simulink model "model_1D_jumpup"  (R2016a)
settings: Solver=FixedStepAuto  StartTime=0.0  StopTime=10.0  FixedStep=deltaT  RelTol=1e-3
undefined symbols (not defined in the file): C_phi, g, l_AB, l_AC, m_K, m_R, O_A_K, phi_0, phi__d_0
settings Model: Creator=ich  LastModifiedBy=ich

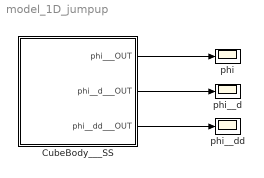
== system model_1D_jumpup ==
  CubeBody___SS : Subsystem
  phi : Scope
  phi__d : Scope
  phi__dd : Scope
  wires:
  CubeBody___SS/3(phi__dd___OUT) -> phi__dd/1
  CubeBody___SS/1(phi___OUT) -> phi/1
  CubeBody___SS/2(phi__d___OUT) -> phi__d/1

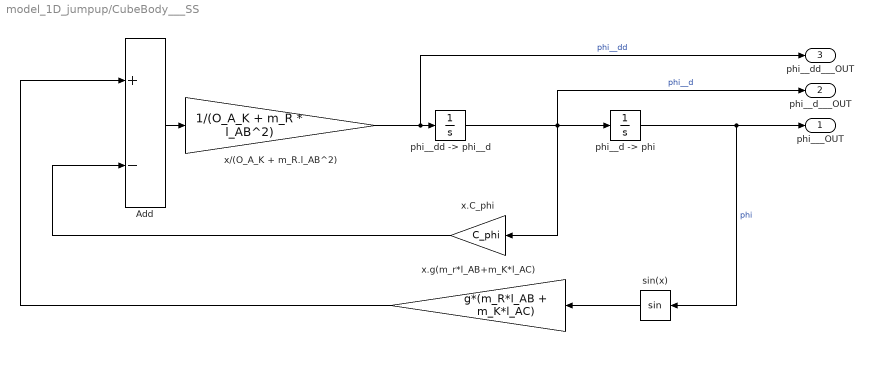
== system model_1D_jumpup/CubeBody___SS ==
  Add : Sum  Inputs=+-
  "phi__d -> phi" : Integrator  InitialCondition=phi_0
  "phi__dd -> phi__d" : Integrator  InitialCondition=phi__d_0
  sin(x) : Trigonometry
  x.C_phi : Gain  Gain=C_phi
  x.g(m_r*l_AB+m_K*l_AC) : Gain  Gain=g*(m_R*l_AB + m_K*l_AC)
  x/(O_A_K + m_R.l_AB^2) : Gain  Gain=1/(O_A_K + m_R * l_AB^2)
  phi___OUT : Outport
  phi__d___OUT : Outport  Port=2
  phi__dd___OUT : Outport  Port=3
  wires:
  "phi__d -> phi"/1 -> sin(x)/1, phi___OUT/1  "phi"
  "phi__dd -> phi__d"/1 -> x.C_phi/1, phi__d___OUT/1, "phi__d -> phi"/1  "phi__d"
  x/(O_A_K + m_R.l_AB^2)/1 -> phi__dd___OUT/1, "phi__dd -> phi__d"/1  "phi__dd"
  Add/1 -> x/(O_A_K + m_R.l_AB^2)/1
  sin(x)/1 -> x.g(m_r*l_AB+m_K*l_AC)/1
  x.g(m_r*l_AB+m_K*l_AC)/1 -> Add/1
  x.C_phi/1 -> Add/2
